simulink model "lqr_controller_with_euler_angle_compensator"  (R2024a)
settings: Solver=VariableStepAuto  StartTime=0.0  StopTime=100  RelTol=1e-3
values from neighbouring files (symbols this model uses):
  lqr1 = lqr(sys,Q,R)    [lqr_quad_for_body_rate_control_model.m]    (also in lqr_quad_for_euler_rate_control_model.m)
  sys = ss(quad_state_A,quad_actuator_B,observer_C,D)    [lqr_quad_for_body_rate_control_model.m]    (also in lqr_quad_for_euler_rate_control_model.m)
libraries: simulink x2
settings Model: SimulationMode=accelerator  Creator=karukkuvelRajDeivasu  LastModifiedBy=karukkuvelRajDeivasu

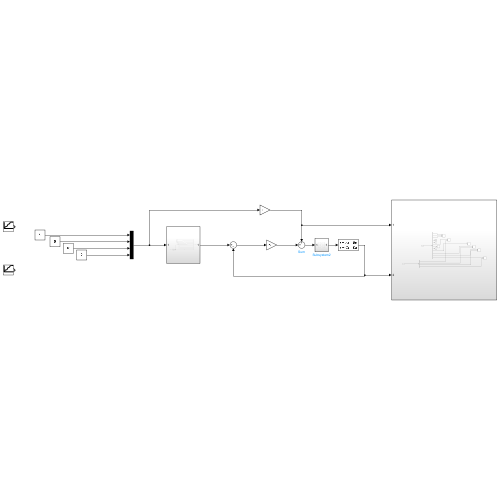
[thumbnail: Simulink's stored preview of the top-level diagram]
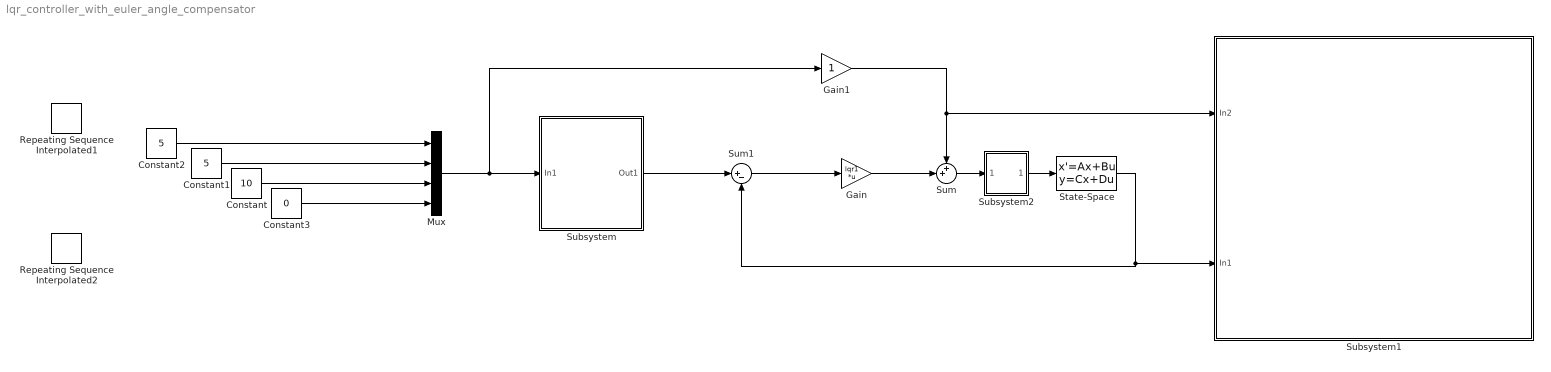
== system lqr_controller_with_euler_angle_compensator ==
  Constant : Constant  Value=10
  Constant1 : Constant  Value=5
  Constant2 : Constant  Value=5
  Constant3 : Constant  Value=0
  Gain : Gain  Gain=lqr1  Multiplication=Matrix(K*u)
  Gain1 : Gain
  Mux : Mux
  Repeating Sequence Interpolated1 : simulink/Sources/Repeating Sequence Interpolated  OutValues=[0 2 2 4 4 6 6 6]  TimeValues=[0 10 20 30 40 50 60 70]/2  LookUpMeth=Interpolation-Use End Values  tsamp=0.001  OutMin=[]  OutMax=[]  OutDataTypeStr=double  OutputDataTypeScalingMode=double  OutDataType=fixdt(0,8)  OutScaling=2^-10
  Repeating Sequence Interpolated2 : simulink/Sources/Repeating Sequence Interpolated  OutValues=[0 2 2 4 4 6 6 6]  TimeValues=[0 10 20 30 40 50 60 70]/2  LookUpMeth=Interpolation-Use End Values  tsamp=0.001  OutMin=[]  OutMax=[]  OutDataTypeStr=double  OutputDataTypeScalingMode=double  OutDataType=fixdt(0,8)  OutScaling=2^-10
  State-Space : StateSpace  A=sys.A  B=sys.B  C=sys.C  D=sys.D  InitialCondition=0
  Subsystem : Subsystem
  Subsystem1 : Subsystem
  Subsystem2 : Subsystem
  Sum : Sum  Inputs=++|
  Sum1 : Sum  Inputs=|+-
  wires:
  State-Space/1 -> Sum1/2, Subsystem1/2(In1)
  Sum1/1 -> Gain/1
  Gain/1 -> Sum/2
  Sum/1 -> Subsystem2/1(In1)
  Subsystem/1(Out1) -> Sum1/1
  Constant1/1 -> Mux/2
  Constant2/1 -> Mux/1
  Constant/1 -> Mux/3
  Mux/1 -> Subsystem/1(In1), Gain1/1
  Constant3/1 -> Mux/4
  Gain1/1 -> Subsystem1/1(In2), Sum/1
  Subsystem2/1(Out1) -> State-Space/1

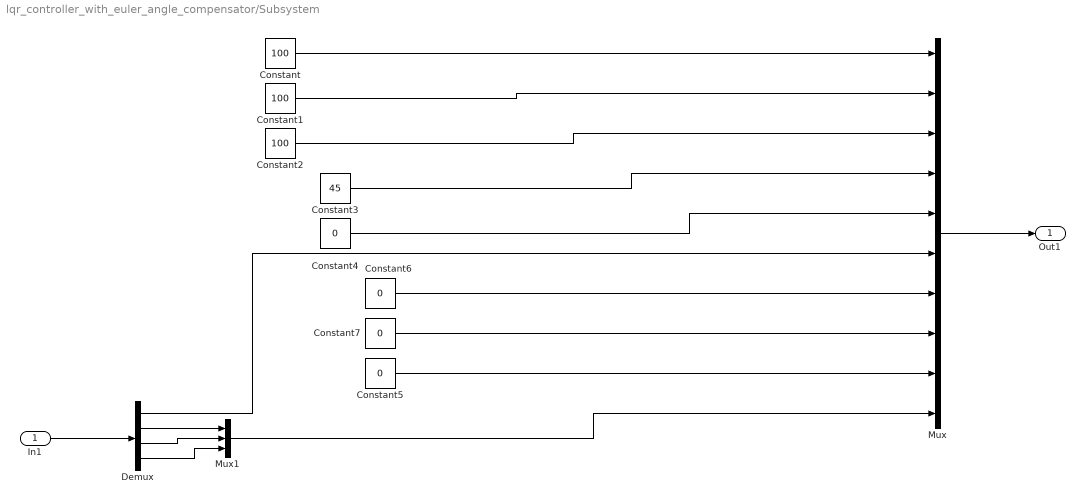
== system lqr_controller_with_euler_angle_compensator/Subsystem ==
  In1 : Inport
  Constant : Constant  Value=100
  Constant1 : Constant  Value=100
  Constant2 : Constant  Value=100
  Constant3 : Constant  Value=45
  Constant{4..7} (4 alike) : Constant  Value=0
  Demux : Demux
  Mux : Mux  Inputs=10
  Mux1 : Mux  Inputs=3
  Out1 : Outport
  wires:
  Mux/1 -> Out1/1
  Constant/1 -> Mux/1
  Constant1/1 -> Mux/2
  Constant2/1 -> Mux/3
  Constant3/1 -> Mux/4
  Constant4/1 -> Mux/5
  Demux/1 -> Mux/6
  Constant6/1 -> Mux/7
  Constant7/1 -> Mux/8
  Constant5/1 -> Mux/9
  Demux/2 -> Mux1/1
  Demux/3 -> Mux1/2
  Demux/4 -> Mux1/3
  Mux1/1 -> Mux/10
  In1/1 -> Demux/1

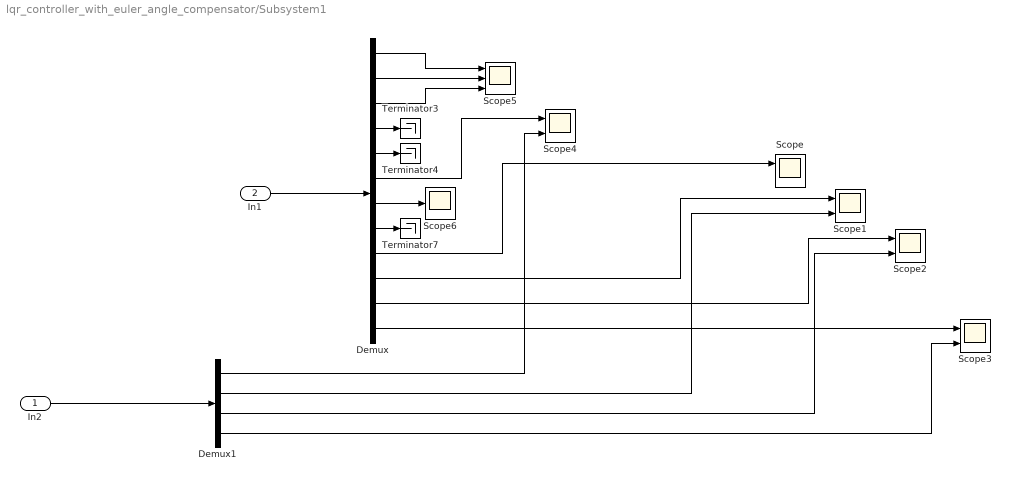
== system lqr_controller_with_euler_angle_compensator/Subsystem1 ==
  In2 : Inport
  In1 : Inport  Port=2
  Demux : Demux  Outputs=12
  Demux1 : Demux
  Scope{,1..4} (5 alike) : Scope  NumInputPorts=2
  Scope5 : Scope  NumInputPorts=3
  Scope6 : Scope
  Terminator3 : Terminator
  Terminator4 : Terminator
  Terminator7 : Terminator
  wires:
  Demux/11 -> Scope2/1
  Demux/9 -> Scope/1
  Demux/12 -> Scope3/1
  Demux/1 -> Scope5/1
  In1/1 -> Demux/1
  Demux/10 -> Scope1/1
  In2/1 -> Demux1/1
  Demux1/1 -> Scope4/2
  Demux1/2 -> Scope1/2
  Demux1/3 -> Scope2/2
  Demux1/4 -> Scope3/2
  Demux/2 -> Scope5/2
  Demux/5 -> Terminator4/1
  Demux/7 -> Scope6/1
  Demux/6 -> Scope4/1
  Demux/8 -> Terminator7/1
  Demux/4 -> Terminator3/1
  Demux/3 -> Scope5/3

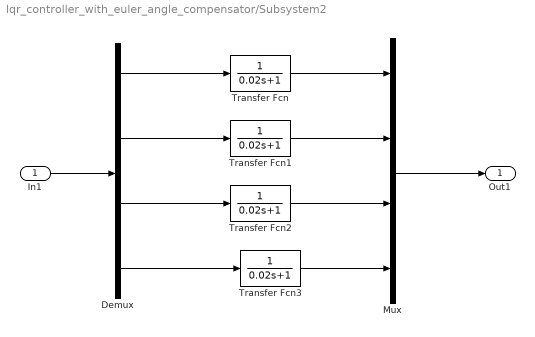
== system lqr_controller_with_euler_angle_compensator/Subsystem2 ==
  In1 : Inport
  Demux : Demux
  Mux : Mux
  Transfer Fcn{,1..3} (4 alike) : TransferFcn  Denominator=[0.02 1]
  Out1 : Outport
  wires:
  In1/1 -> Demux/1
  Demux/1 -> Transfer Fcn/1
  Demux/2 -> Transfer Fcn1/1
  Demux/3 -> Transfer Fcn2/1
  Demux/4 -> Transfer Fcn3/1
  Transfer Fcn/1 -> Mux/1
  Transfer Fcn1/1 -> Mux/2
  Transfer Fcn2/1 -> Mux/3
  Transfer Fcn3/1 -> Mux/4
  Mux/1 -> Out1/1
